simulink model "demo1"  (R2024b)
settings: Solver=FixedStepAuto  StartTime=0.0  StopTime=T  FixedStep=dt  RelTol=1e-3
values from neighbouring files (symbols this model uses):
  alp = opt.alpha    [demo1_src.m]
  beta = opt.beta    [demo1_src.m]
  ctrl_dt = 1/250    (= 0.004)    [demo1_src.m]
  Lambda = opt.Lambda    [demo1_src.m]
  lbd = zeros(4, 1)    [demo1_src.m]
  th = (rand(opt.th_size,1)-1/2)*2*opt.init_range    [demo1_src.m]
  th_max = opt.cstr.th_max    [demo1_src.m]
  u_ball = opt.cstr.u_ball    [demo1_src.m]
  x1 = [deg2rad(-90);0]    [demo1_src.m]
  x2 = [0;0]    [demo1_src.m]
undefined symbols (not defined in the file or in its folder): ctrl, nnOpt, zeta
settings Model: Creator=dding  LastModifiedBy=dding
settings OptimizationCC: ReuseModelBlockBuffer=off
settings RTWCC: GPUComputeCapability=3.5

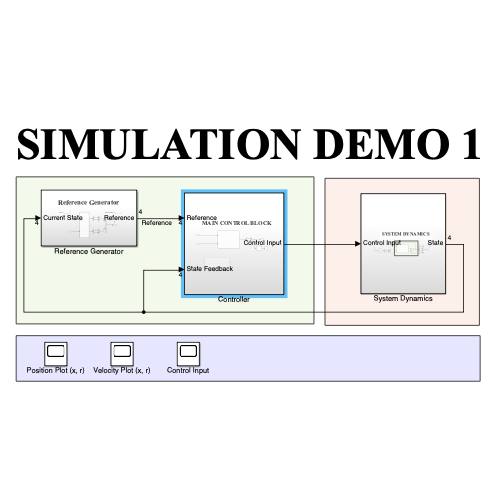
[thumbnail: Simulink's stored preview of the top-level diagram]
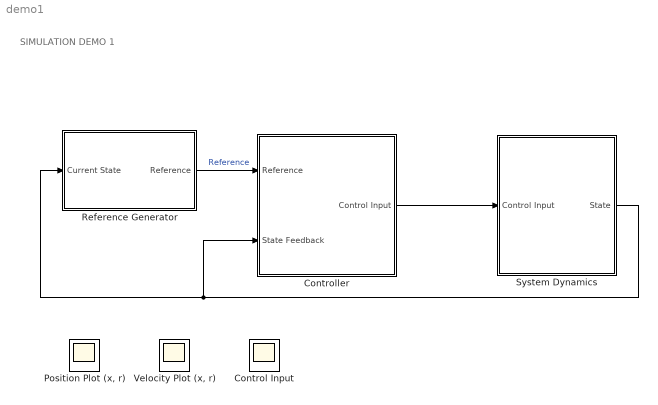
== system demo1 ==
  note: SIMULATION DEMO 1
  Control Input : Scope
      settings: Floating=on
  Controller : Subsystem
  "Position Plot (x, r)" : Scope
      settings: Floating=on
  Reference Generator : Subsystem
  System Dynamics : Subsystem
  "Velocity Plot (x, r)" : Scope
      settings: Floating=on
  wires:
  System Dynamics/1(State) -> Reference Generator/1(Current State), Controller/2(State Feedback)
  Reference Generator/1(Reference) -> Controller/1(Reference)  "Reference"
  Controller/1(Control Input) -> System Dynamics/1(Control Input)

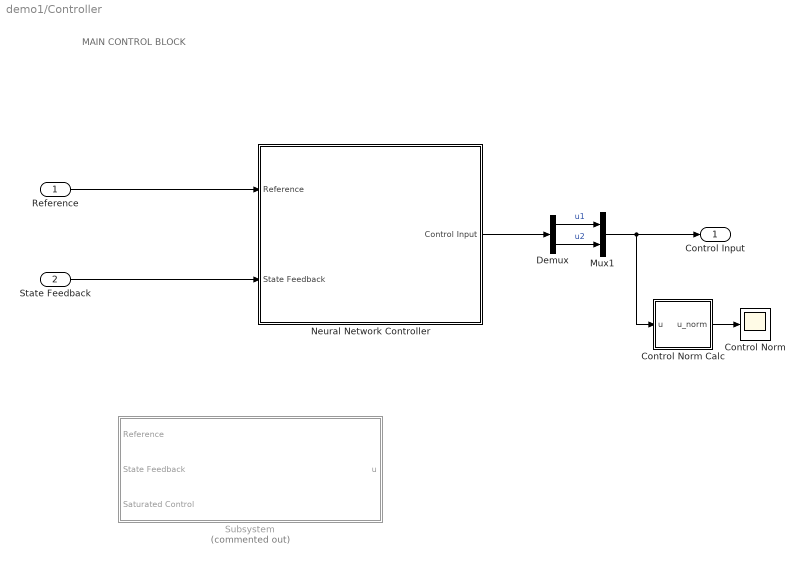
== system demo1/Controller ==
  note: MAIN CONTROL BLOCK
  Reference : Inport
  State Feedback : Inport  Port=2
  Control Norm : Scope
  Control Norm Calc : MATLAB Function  TreatAsAtomicUnit=on
  Demux : Demux  Outputs=2
  Mux1 : Mux  Inputs=2
  Neural Network Controller : Subsystem
  Subsystem : Subsystem  Commented=on
  Control Input : Outport
  wires:
  Reference/1 -> Neural Network Controller/1(Reference)
  State Feedback/1 -> Neural Network Controller/2(State Feedback)
  Demux/2 -> Mux1/2  "u2"
  Demux/1 -> Mux1/1  "u1"
  Mux1/1 -> Control Norm Calc/1(u), Control Input/1
  Control Norm Calc/1(u_norm) -> Control Norm/1
  Neural Network Controller/1(Control Input) -> Demux/1

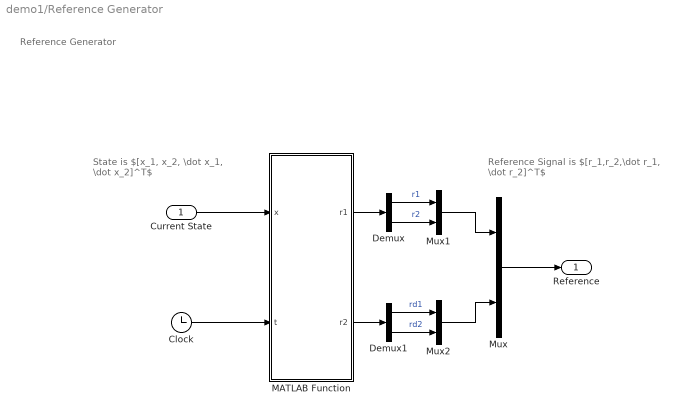
== system demo1/Reference Generator ==
  note: Reference Signal is $[r_1,r_2,\dot r_1, \dot r_2]^T$
  note: Reference Generator
  note: State is $[x_1, x_2, \dot x_1, \dot x_2]^T$
  Current State : Inport
  Clock : Clock
  Demux : Demux  Outputs=2
  Demux1 : Demux  Outputs=2
  MATLAB Function : MATLAB Function  TreatAsAtomicUnit=on
  Mux : Mux  Inputs=2
  Mux1 : Mux  Inputs=2
  Mux2 : Mux  Inputs=2
  Reference : Outport
  wires:
  Current State/1 -> MATLAB Function/1(x)
  Clock/1 -> MATLAB Function/2(t)
  MATLAB Function/1(r1) -> Demux/1
  Mux/1 -> Reference/1
  Demux/1 -> Mux1/1  "r1"
  Demux/2 -> Mux1/2  "r2"
  Mux1/1 -> Mux/1
  Demux1/2 -> Mux2/2  "rd2"
  Demux1/1 -> Mux2/1  "rd1"
  MATLAB Function/2(r2) -> Demux1/1
  Mux2/1 -> Mux/2

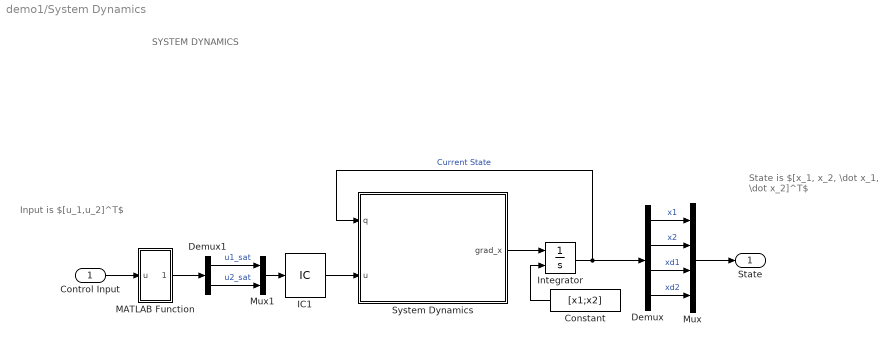
== system demo1/System Dynamics ==
  note: SYSTEM DYNAMICS
  note: State is $[x_1, x_2, \dot x_1, \dot x_2]^T$
  note: Input is $[u_1,u_2]^T$
  Control Input : Inport
  Constant : Constant  Value=[x1;x2]
  Demux : Demux
  Demux1 : Demux  Outputs=2
  IC1 : InitialCondition  Value=[0; 0];
  Integrator : Integrator  InitialConditionSource=external
  MATLAB Function : MATLAB Function  TreatAsAtomicUnit=on
  Mux : Mux
  Mux1 : Mux  Inputs=2
  System Dynamics : MATLAB Function  TreatAsAtomicUnit=on
  State : Outport
  wires:
  Control Input/1 -> MATLAB Function/1(u)
  System Dynamics/1(grad_x) -> Integrator/1
  Integrator/1 -> Demux/1, System Dynamics/1(q)  "Current State"
  IC1/1 -> System Dynamics/2(u)
  Constant/1 -> Integrator/2
  Mux/1 -> State/1
  Demux/1 -> Mux/1  "x1"
  Demux/2 -> Mux/2  "x2"
  Demux/3 -> Mux/3  "xd1"
  Demux/4 -> Mux/4  "xd2"
  MATLAB Function/1(u_sat) -> Demux1/1
  Demux1/1 -> Mux1/1  "u1_sat"
  Demux1/2 -> Mux1/2  "u2_sat"
  Mux1/1 -> IC1/1

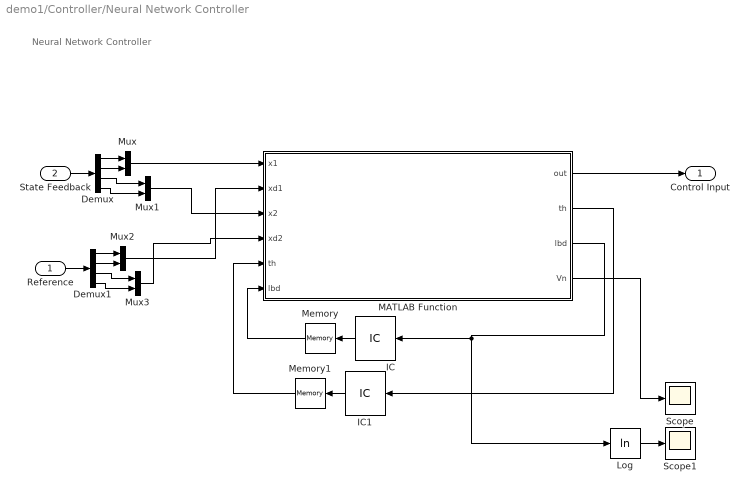
== system demo1/Controller/Neural Network Controller ==
  note: Neural Network Controller
  Reference : Inport
  State Feedback : Inport  Port=2
  Demux : Demux
  Demux1 : Demux
  IC : InitialCondition  Value=lbd
  IC1 : InitialCondition  Value=th
  Log : Math  Operator=log
  MATLAB Function : MATLAB Function  TreatAsAtomicUnit=on  SystemSampleTime=ctrl_dt
  Memory : Memory
  Memory1 : Memory
  Mux{,1..3} (4 alike) : Mux  Inputs=2
  Scope : Scope
  Scope1 : Scope
  Control Input : Outport
  wires:
  MATLAB Function/1(out) -> Control Input/1
  MATLAB Function/4(Vn) -> Scope/1
  IC/1 -> Memory/1
  IC1/1 -> Memory1/1
  State Feedback/1 -> Demux/1
  Demux/1 -> Mux/1
  Demux/2 -> Mux/2
  Mux/1 -> MATLAB Function/1(x1)
  Demux/3 -> Mux1/1
  Demux/4 -> Mux1/2
  Mux1/1 -> MATLAB Function/3(x2)
  Mux3/1 -> MATLAB Function/4(xd2)
  Demux1/4 -> Mux3/2
  Demux1/3 -> Mux3/1
  Mux2/1 -> MATLAB Function/2(xd1)
  Demux1/2 -> Mux2/2
  Demux1/1 -> Mux2/1
  Reference/1 -> Demux1/1
  MATLAB Function/2(th) -> IC1/1
  MATLAB Function/3(lbd) -> Log/1, IC/1
  Memory/1 -> MATLAB Function/6("lbd ")
  Memory1/1 -> MATLAB Function/5("th ")
  Log/1 -> Scope1/1

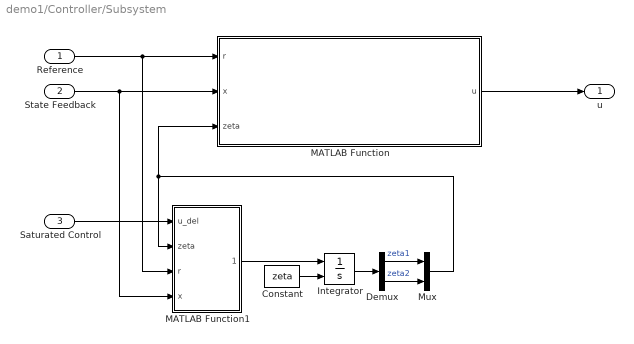
== system demo1/Controller/Subsystem ==
  Reference : Inport
  State Feedback : Inport  Port=2
  Saturated Control : Inport  Port=3
  Constant : Constant  Value=zeta
  Demux : Demux  Outputs=2
  Integrator : Integrator  InitialConditionSource=external
  MATLAB Function : MATLAB Function  TreatAsAtomicUnit=on
  MATLAB Function1 : MATLAB Function  TreatAsAtomicUnit=on
  Mux : Mux  Inputs=2
  u : Outport
  wires:
  MATLAB Function/1(u) -> u/1
  State Feedback/1 -> MATLAB Function1/4(x), MATLAB Function/2(x)
  Reference/1 -> MATLAB Function1/3(r), MATLAB Function/1(r)
  Constant/1 -> Integrator/2
  Saturated Control/1 -> MATLAB Function1/1(u_del)
  MATLAB Function1/1(grad_zeta) -> Integrator/1
  Integrator/1 -> Demux/1
  Demux/1 -> Mux/1  "zeta1"
  Demux/2 -> Mux/2  "zeta2"
  Mux/1 -> MATLAB Function1/2(zeta), MATLAB Function/3(zeta)

== matlab function demo1/Reference Generator/MATLAB Function ==
  data: x input; r1 output; t input; r2 output
function [r1, r2] = fcn(x, t)

x0 = [deg2rad(-90);0];  
xd = [0;deg2rad(30)];
% xd = [0;deg2rad(10)];
T = 3;    

t = mod(t, 2*T);

if t < T
    [r1,r2] = poly_filter(x0, xd, T, t);
else
    [r1,r2] = poly_filter(xd, x0, T, (t-T));
end

end

function [r1, r2] = poly_filter(x0, xd, T, t)

a0 = x0;
a1 = zeros(2,1);
a2 = zeros(2,1);
a3 = 10*(xd-a0)/T^3;
a4 = -15*(xd-x0)/T^4;
a5 = 6*(xd-a0)/T^5;

r1 = [a0 a1 a2 a3 a4 a5] * [1 t t^2 t^3 t^4 t^5]';
r2 = [a1 a2 a3 a4 a5] * [1 2*t 3*t^2 4*t^3 5*t^4]';

end

== matlab function demo1/System Dynamics/System Dynamics ==
  data: q input; u input; grad_x output
function grad_x = fcn(q, u)

%% SYSTEM DYNAMICS
grad_x = model_wrapper(q, u, 0);

end

function f = model_wrapper(q, u, t)
    [M, C, G, F ] = model1(q, t);
    
    del_M = zeros(2,2); 
    % del_C = [
    %     tanh(q(1))*100
    %     -tanh(q(2))*100
    % ]; 
    del_C = zeros(2,2); 

    % del_G = rand(2,1)*1e0;
    del_G = zeros(2,1);

    M = M + del_M;
    C = C + del_C;
    G = G + del_G;

    % d = [
    %     tanh(q(1))*20 + sin(5*t)*3e1
    %     -tanh(q(2))*20 + cos(5*t)*3e1
    % ];
    d = zeros(2,1);

    f1 = q(3:4);
    f2 = M \ (-C*q(3:4) -G -F +u +d);
    
    f = [f1 ; f2];
end

function [M, C, G, F, J] = model1(q, t)
% 2 link manipulator dynamics

%% Parameters
% ********************************************************

m1 = 2.465;             % [kg]
m2 = 1.093;
L1 = .2;             % [m]
L2 = .15+.01+.02;
Lc1 = .13888;             % [m]
Lc2 = .08691;
g = 9.81;             % [m/s^2]

b1 = .2;
b2 = .1;
fc1 = .35;
fc2 = .2;

I1 = .06911;
I2 = .01532;

%%
q1 = q(1); q2 = q(2);

qd = q(3:4);
qd1 = qd(1); qd2 = qd(2); 

%%
Mmat11=I1+I2+Lc1^2*m1+L1^2*m2+Lc2^2*m2+2*L1*Lc2*m2*cos(q2);
Mmat12=I2+Lc2^2*m2+L1*Lc2*m2*cos(q2);
Mmat21=I2+Lc2^2*m2+L1*Lc2*m2*cos(q2);
Mmat22=I2+Lc2^2*m2;
Cmat11=(-1)*L1*Lc2*m2*sin(q2)*qd2;
Cmat12=(-1)*L1*Lc2*m2*sin(q2)*(qd1+qd2);
Cmat21=L1.*Lc2*m2*sin(q2)*qd1;
Cmat22=0;
Gmat1=g*((Lc1*m1+L1*m2)*cos(q1)+Lc2*m2*cos(q1+q2));
Gmat2=g*Lc2*m2*cos(q1+q2);
Fmat1=b1*sign(qd1)+fc1*qd1;
Fmat2=b2*sign(qd2)+fc2*qd2;
Jmat11 = (-1).*L1.*sin(q1)+(-1).*L2.*sin(q1+q2); 
Jmat12 = (-1).*L2.*sin(q1+q2);
Jmat21 = L1.*cos(q1)+L2.*cos(q1+q2); 
Jmat22 = L2.*cos(q1+q2);

%%
M = [
    Mmat11 Mmat12
    Mmat21 Mmat22  
    ];
C = [
    Cmat11 Cmat12
    Cmat21 Cmat22  
    ];
G = [
    Gmat1
    Gmat2
    ];
F = [
    Fmat1
    Fmat2
    ];
J = [
    Jmat11 Jmat12
    Jmat21 Jmat22
    ];

end

== matlab function demo1/Controller/Neural Network Controller/MATLAB Function ==
  data: x1 input; out output; xd1 input; x2 input; xd2 input; th input; lbd input; th output; lbd output; Vn output; alp parameter; ctrl_dt parameter; Lambda parameter; th_max parameter; u_ball parameter; beta parameter
function [out, th, lbd, Vn] = CoNAC(x1, xd1, x2, xd2, th, lbd, alp, ctrl_dt, Lambda, th_max, u_ball, beta)
    %% Parameters
    NN_size = [
            % layer info (node numbers)
            6 % input layer
            4
            4
            2 % output layer
    ]; 
    l_size = length(NN_size); 
    tp_size = sum(NN_size(1:end-1)); 
    th_size_list = zeros(l_size-1 ,1); 

    for idx = 1:l_size-1
        th_size_list(idx) = (NN_size(idx) + 1) * NN_size(idx + 1);      
    end
    th_size = sum(th_size_list); 
    lbd_size = l_size-1 + 1; % multiplier number

    %% FEEDFORWAD 
    % ================================================
    %     FEEDFORWARD (CONTROL INPUT CALCULATION)
    % ================================================
    pt_V = 1;
    Vn = zeros(l_size-1, 1);

    % neural network input
    e1 = x1-xd1; e2 = x2-xd2;
    e = e2+Lambda*e1;

    in = [x1;xd1;e]; 

    %% FORWARD (layer 1)
    n = NN_size(1)+1;
    m = NN_size(2);

    V0 = zeros(n,m);
    th_index = pt_V;
    for j = 1:m
        for i = 1:n
            V0(i,j) = th(th_index);
            th_index = th_index +1;
        end
    end
    in0 = [in; 1];

    out0 = V0'*in0;

    % pointer to next
    pt_V = pt_V + (n*m);

    % current norm
    Vn(1) = norm(V0);

    %% FORWARD (layer 2)
    n = NN_size(2)+1;
    m = NN_size(3);

    V1 = zeros(n,m);
    th_index = pt_V;
    for j = 1:m
        for i = 1:n
            V1(i,j) = th(th_index);
            th_index = th_index +1;
        end
    end
    in1 = [tanh(out0); 1];

    out1 = V1'*in1;

    % pointer to next
    pt_V = pt_V + (n*m);

    % current norm
    Vn(2) = norm(V1);

    %% FORWARD (layer 3)
    n = NN_size(3)+1;
    m = NN_size(4);

    V2 = zeros(n,m);
    th_index = pt_V;
    for j = 1:m
        for i = 1:n
            V2(i,j) = th(th_index);
            th_index = th_index +1;
        end
    end
    in2 = [tanh(out1); 1];

    out2 = V2'*in2;

    % pointer to next
    pt_V = pt_V + (n*m);

    % current norm
    Vn(3) = norm(V2);
    
    %% RESULT
    assert(pt_V-1 == th_size)
    
    out = out2;

    %% DEAD-ZONE
    % ================================================
    %                   STOP UPDATE
    % ================================================
    % if norm(e) < e_tol
    %     th_grad = zeros(th_size, 1);
    %     lbd_grad = zeros(lbd_size, 1);
    %     return;
    % end

    %% NN GRADIENT CALCULATION
    % ================================================
    %       NEURAL NETWORK JACOBIAN CALCULATION
    % ================================================
    pt_V = th_size;
    pt_tape = tp_size;

    grad_to_back1 = 1;

    %% BACKPROPAGATION (layer end-0)
    l_idx = l_size;
    
    l2 = NN_size(l_idx);        
    l1 = NN_size(l_idx-1);        

    % (I \otimes phi_k^T)
    grad0 = kron(eye(l2), in2');

    %% BACKPROPAGATION (layer end-1)
    l_idx = l_size-1;
      
    l2 = NN_size(l_idx);        
    l1 = NN_size(l_idx-1);          

    grad1 = kron(eye(l2), in1');

    phi_dot1 = tanh_dot(out1);

    grad_to_back1 = grad_to_back1 * V2'*phi_dot1;


    grad1 = grad_to_back1*grad1;
    
    %% BACKPROPAGATION (layer end-2)
    l_idx = l_size-2;
      
    l2 = NN_size(l_idx);        
    l1 = NN_size(l_idx-1);   

    grad2 = kron(eye(l2), in0');

    phi_dot2 = tanh_dot(out0);

    grad_to_back1 = grad_to_back1 * V1'*phi_dot2;

    grad2 = grad_to_back1*grad2;

    %% RESULT
    nnGrad = [grad2 grad1 grad0];

    % ERROR CHECK
    % assert(pt_V == (NN_size(1)+1)*NN_size(2));
    % assert(pt_tape == 0);

    %% CONSTRINT HANDLING
    % ================================================
    %     
    % ================================================

    %% CONSTRAINT FUNC. CALCULATION
    % ball condition 
    cumsum_V = [0;cumsum(th_size_list)];
    c_b = Vn.^2 - th_max.^2;

    % input ball 
    c_ub = norm(out)^2 - u_ball^2;
    
    % summary
    c = [c_b; c_ub];

    %% CONSTRAINT GREADIENT (dC/dth)
    cd = zeros(lbd_size, th_size);

    for l_idx = 1:1:length(th_max)
        start_pt = cumsum_V(l_idx)+1;
        end_pt = cumsum_V(l_idx+1);

        cd(l_idx, start_pt:end_pt) = 2 * th(start_pt:end_pt,1);
    end
    
    cd(l_idx+1:end, :) = 2*nnGrad'*out;
 
    %% BACKPROPAGATION 
    % ================================================
    %     BACKPROPAGATION (NEURAL NETWROK UPDATE)
    % ================================================
    th_grad = -alp*nnGrad'*e; % dJ/dth
    th_grad = th_grad - alp* cd' * lbd; % dC/dth

    lbd_grad = diag(beta) * c;

    th = th + th_grad * ctrl_dt;
    lbd = lbd + lbd_grad * ctrl_dt;
    lbd = max(lbd, 0);

    return
end

%% LOCAL FUNCTIONS
function phi_dot = tanh_dot(Phi)
    phi_dot = zeros(length(Phi)+1, length(Phi));
    for idx = 1:1:length(Phi)
        phi_dot(idx,idx) = 1-tanh(Phi(idx))^2;
    end
end

== matlab function demo1/Controller/Subsystem/MATLAB Function ==
  data: r input; u output; x input; zeta input; nnOpt parameter; ctrl parameter
function u = fcn(r, x, zeta, nnOpt, ctrl)
%%
e = x - r(1:4);
e1 = e(1:2);
e2 = e(3:4);
r2d = r(5:6);

%%
k2 = nnOpt.ctrl_param.k2;
Kp = nnOpt.ctrl_param.Kp;
M = nnOpt.ctrl_param.M;
C = nnOpt.ctrl_param.C;
G = nnOpt.ctrl_param.G;

%% ALGORITHM PARAMETERS

%% control input
if ctrl == 1
    u = -M*k2*e2 -M*e1 + C*x(3:4) + G +M*r2d;

elseif ctrl == 2 
    u1 = - M * k2 * e2 - M * e1 + C * x(3:4) + G + M * r2d;
    u2 = - M * Kp * zeta;

    u = u1 + u2;
    % u = u1;

elseif ctrl == 3
    u1 = - M * k2 * e2 - M * e1 + C * x(3:4) + G + M * r2d;
    u2 = + M * Kp * zeta;

    u = u1 + u2;
    % u = u1;

elseif ctrl == 4
    u = zeros(2,1);
else 
    u = zeros(2,1);

end

== matlab function demo1/Controller/Control Norm Calc ==
  data: u input; u_norm output
function u_norm = fcn(u)

u_norm = norm(u);

end

== matlab function demo1/System Dynamics/MATLAB Function ==
  data: u input; u_sat output; u_ball parameter
function u_sat = fcn(u, u_ball)
    if norm(u) > u_ball
        u_sat = u/norm(u) * u_ball;
    else
        u_sat = u;
    end
end

== matlab function demo1/Controller/Subsystem/MATLAB Function1 ==
  data: u_del input; grad_zeta output; zeta input; r input; x input; nnOpt parameter
function grad_zeta = fcn(u_del, zeta, r, x, nnOpt)

%%
e = x - r(1:4);
e2 = e(3:4);

%%
Azeta = nnOpt.ctrl_param.Azeta;
% nnOpt.ctrl_param.Bzeta;
mu = nnOpt.ctrl_param.mu;

%%
if norm(zeta) >= mu
    grad_zeta = -Azeta * zeta ...
        - (( abs(e2'*u_del) +0.5*(u_del'*u_del) )/norm(zeta)^2) *zeta ...        
        + u_del;
else
    grad_zeta = zeros(size(zeta));
end

end
